simulink model "Motor_Model_lag"  (R2025b)
settings: Solver=ode45  StartTime=0.0  StopTime=2  RelTol=1e-3
undefined symbols (not defined in the file): b, J, K, L, R
settings Model: Creator=sansh  LastModifiedBy=sjawahar
settings SolverCC: AlgebraicLoopSolver=TrustRegion
settings DataIOCC: ReturnWorkspaceOutputs=off
settings DebuggingCC: UnconnectedInputMsg=warning  UnconnectedOutputMsg=warning  UnconnectedLineMsg=warning  ArithmeticOperatorsInVariantConditions=warning
settings ModelReferenceCC: EnableRefExpFcnMdlSchedulingChecks=on
settings SFSimCC: SimUseLocalCustomCode=off  CustomCodeUndefinedFunction=UseInterfaceOnly
settings RTWCC: RTWUseLocalCustomCode=off  GPUComputeCapability=3.5
settings CodeAppCC: StateflowObjectComments=on

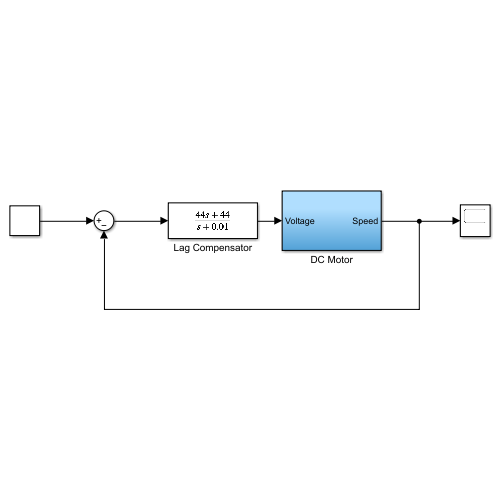
[thumbnail: Simulink's stored preview of the top-level diagram]
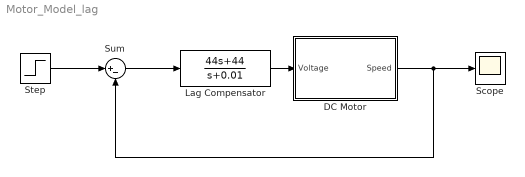
== system Motor_Model_lag ==
  DC Motor : Subsystem
  Lag Compensator : TransferFcn  Numerator=[44 44]  Denominator=[1 0.01]
  Scope : Scope
      settings: ActiveDisplayYMinimum=-0.01245  ActiveDisplayYMaximum=0.11204
  Step : Step  Time=0  SampleTime=0
  Sum : Sum  Inputs=|+-
  wires:
  DC Motor/1(Speed) -> Sum/2, Scope/1
  Step/1 -> Sum/1
  Sum/1 -> Lag Compensator/1
  Lag Compensator/1 -> DC Motor/1(Voltage)

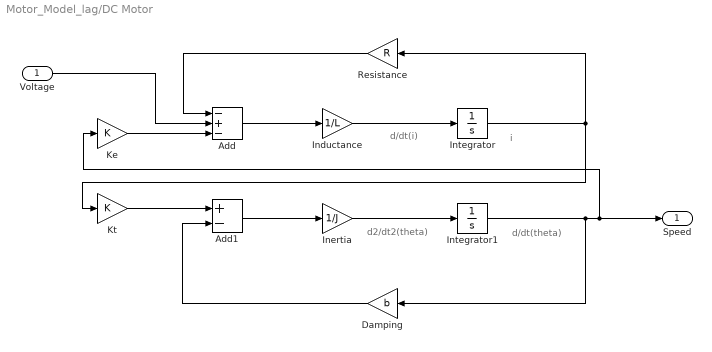
== system Motor_Model_lag/DC Motor ==
  note: i
  note: d/dt(i)
  note: d/dt(theta)
  note: d2/dt2(theta)
  Voltage : Inport
  Add : Sum  Inputs=-+-
  Add1 : Sum  Inputs=+-
  Damping : Gain  Gain=b
  Inductance : Gain  Gain=1/L
  Inertia : Gain  Gain=1/J
  Integrator : Integrator
  Integrator1 : Integrator
  Ke : Gain  Gain=K
  Kt : Gain  Gain=K
  Resistance : Gain  Gain=R
  Speed : Outport
  wires:
  Inductance/1 -> Integrator/1
  Integrator1/1 -> Damping/1, Speed/1, Ke/1
  Inertia/1 -> Integrator1/1
  Integrator/1 -> Resistance/1, Kt/1
  Kt/1 -> Add1/1
  Voltage/1 -> Add/2
  Resistance/1 -> Add/1
  Damping/1 -> Add1/2
  Ke/1 -> Add/3
  Add/1 -> Inductance/1
  Add1/1 -> Inertia/1
